simulink model "Engine_Propeller_Model_SAAM"  (R2018a)
settings: Solver=FixedStepAuto  StartTime=0.0  StopTime=10.0  FixedStep=dt  RelTol=1e-3
values from neighbouring files (symbols this model uses):
  dt = 0.05    [SmallAerobaticAirplaneModel.m]    (also in motorSpeedSS.m = 1; trim_airplane_min.m = 0.01)
  motorSpeed0 = 0    [SmallAerobaticAirplaneModel.m]    (also in create_engine_tables.m = fmincon(@(x)motorSpeedSS(x, Up, Vp, Wp, airDens, P_e_ic, vi0; trim_airplane_min.m = fmincon(@(x)motorSpeedSS(x, vcaso*cosd(aoadic), 0, -vcaso*si)
  vi0 = vcas(1)    [SmallAerobaticAirplaneModel.m]    (also in calculateThrustState.m = 0.001; create_engine_tables.m = fsolve(@(x)findVi2(x, vcaso*cosd(aoadic), 0, -vcaso*sind(aoa; findThrust.m = 0.01; trim_airplane_min.m = fsolve(@(x)findVi2(x, vcaso*cosd(aoadic), 0, -vcaso*sind(aoa)
settings Model: Creator=Kyle  LastModifiedBy=Kyle

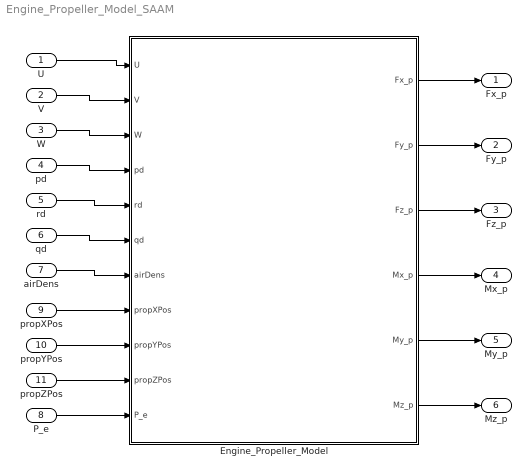
== system Engine_Propeller_Model_SAAM ==
  U : Inport
  V : Inport  Port=2
  W : Inport  Port=3
  pd : Inport  Port=4
  rd : Inport  Port=5
  qd : Inport  Port=6
  airDens : Inport  Port=7
  P_e : Inport  Port=8
  propXPos : Inport  Port=9
  propYPos : Inport  Port=10
  propZPos : Inport  Port=11
  Engine_Propeller_Model : Subsystem
  Fx_p : Outport
  Fy_p : Outport  Port=2
  Fz_p : Outport  Port=3
  Mx_p : Outport  Port=4
  My_p : Outport  Port=5
  Mz_p : Outport  Port=6
  wires:
  U/1 -> Engine_Propeller_Model/1(U)
  V/1 -> Engine_Propeller_Model/2(V)
  W/1 -> Engine_Propeller_Model/3(W)
  pd/1 -> Engine_Propeller_Model/4(pd)
  propXPos/1 -> Engine_Propeller_Model/8(propXPos)
  propYPos/1 -> Engine_Propeller_Model/9(propYPos)
  propZPos/1 -> Engine_Propeller_Model/10(propZPos)
  P_e/1 -> Engine_Propeller_Model/11(P_e)
  rd/1 -> Engine_Propeller_Model/5(rd)
  qd/1 -> Engine_Propeller_Model/6(qd)
  airDens/1 -> Engine_Propeller_Model/7(airDens)
  Engine_Propeller_Model/4(Mx_p) -> Mx_p/1
  Engine_Propeller_Model/6(Mz_p) -> Mz_p/1
  Engine_Propeller_Model/5(My_p) -> My_p/1
  Engine_Propeller_Model/2(Fy_p) -> Fy_p/1
  Engine_Propeller_Model/1(Fx_p) -> Fx_p/1
  Engine_Propeller_Model/3(Fz_p) -> Fz_p/1

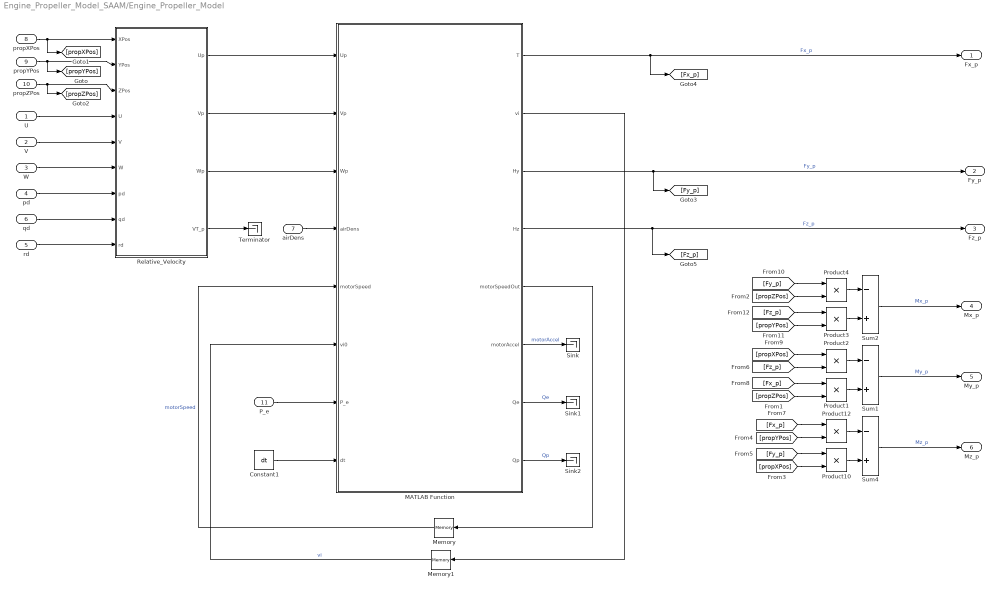
== system Engine_Propeller_Model_SAAM/Engine_Propeller_Model ==
  U : Inport
  V : Inport  Port=2
  W : Inport  Port=3
  pd : Inport  Port=4
  rd : Inport  Port=5
  qd : Inport  Port=6
  airDens : Inport  Port=7
  propXPos : Inport  Port=8
  propYPos : Inport  Port=9
  propZPos : Inport  Port=10
  P_e : Inport  Port=11
  Constant1 : Constant  Value=dt
  MATLAB Function : MATLAB Function  TreatAsAtomicUnit=on
  Memory : Memory  InitialCondition=motorSpeed0  LinearizeAsDelay=on
  Memory1 : Memory  InitialCondition=vi0  LinearizeAsDelay=on
  Product{1..4,10,12} (6 alike) : Product
  Relative_Velocity : Subsystem
  Sink : Terminator
  Sink1 : Terminator
  Sink2 : Terminator
  Sum1 : Sum  Inputs=-+
  Sum2 : Sum  Inputs=-+
  Sum4 : Sum  Inputs=-+
  Terminator : Terminator
  Fx_p : Outport
  Fy_p : Outport  Port=2
  Fz_p : Outport  Port=3
  Mx_p : Outport  Port=4
  My_p : Outport  Port=5
  Mz_p : Outport  Port=6
  wires:
  propYPos/1 -> [propYPos], Relative_Velocity/2(YPos)
  propZPos/1 -> [propZPos], Relative_Velocity/3(ZPos)
  U/1 -> Relative_Velocity/4(U)
  V/1 -> Relative_Velocity/5(V)
  W/1 -> Relative_Velocity/6(W)
  pd/1 -> Relative_Velocity/7(pd)
  rd/1 -> Relative_Velocity/9(rd)
  qd/1 -> Relative_Velocity/8(qd)
  propXPos/1 -> [propXPos], Relative_Velocity/1(XPos)
  [propZPos] -> Product1/2
  Product12/1 -> Sum4/1
  Sum4/1 -> Mz_p/1  "Mz_p"
  MATLAB Function/4(Hz) -> [Fz_p], Fz_p/1  "Fz_p"
  [propYPos] -> Product12/2
  Product10/1 -> Sum4/2
  [propXPos] -> Product10/2
  Relative_Velocity/4(VT_p) -> Terminator/1
  Relative_Velocity/1(Up) -> MATLAB Function/1(Up)
  Relative_Velocity/2(Vp) -> MATLAB Function/2(Vp)
  Relative_Velocity/3(Wp) -> MATLAB Function/3(Wp)
  airDens/1 -> MATLAB Function/4(airDens)
  MATLAB Function/5(motorSpeedOut) -> Memory/1
  Memory/1 -> MATLAB Function/5(motorSpeed)  "motorSpeed"
  MATLAB Function/2(vi) -> Memory1/1
  Memory1/1 -> MATLAB Function/6(vi0)  "vi"
  Constant1/1 -> MATLAB Function/8(dt)
  MATLAB Function/1(T) -> [Fx_p], Fx_p/1  "Fx_p"
  MATLAB Function/3(Hy) -> [Fy_p], Fy_p/1  "Fy_p"
  P_e/1 -> MATLAB Function/7(P_e)
  MATLAB Function/6(motorAccel) -> Sink/1  "motorAccel"
  MATLAB Function/7(Qe) -> Sink1/1  "Qe"
  MATLAB Function/8(Qp) -> Sink2/1  "Qp"
  [propZPos] -> Product4/2
  [Fy_p] -> Product10/1
  [Fx_p] -> Product12/1
  Product1/1 -> Sum1/2
  Product2/1 -> Sum1/1
  Sum1/1 -> My_p/1  "My_p"
  [Fx_p] -> Product1/1
  [Fz_p] -> Product2/2
  [propXPos] -> Product2/1
  Product4/1 -> Sum2/1
  Sum2/1 -> Mx_p/1  "Mx_p"
  Product3/1 -> Sum2/2
  [Fy_p] -> Product4/1
  [propYPos] -> Product3/2
  [Fz_p] -> Product3/1

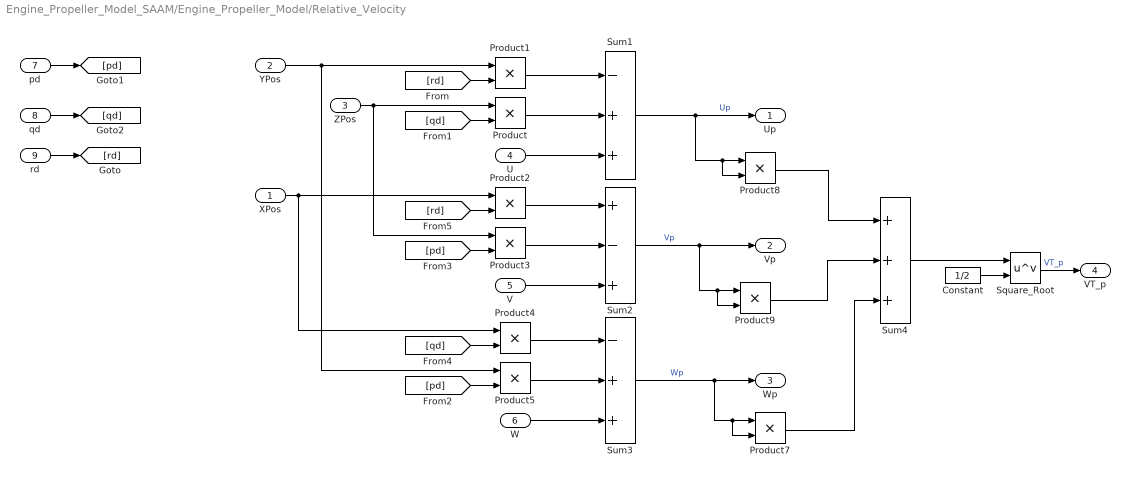
== system Engine_Propeller_Model_SAAM/Engine_Propeller_Model/Relative_Velocity ==
  XPos : Inport
  YPos : Inport  Port=2
  ZPos : Inport  Port=3
  U : Inport  Port=4
  V : Inport  Port=5
  W : Inport  Port=6
  pd : Inport  Port=7
  qd : Inport  Port=8
  rd : Inport  Port=9
  Constant : Constant  Value=1/2
  Product{,1..5,7..9} (9 alike) : Product
  Square_Root : Math  Operator=pow  SaturateOnIntegerOverflow=on
  Sum1 : Sum  Inputs=-++
  Sum2 : Sum  Inputs=+-+
  Sum3 : Sum  Inputs=-++
  Sum4 : Sum  Inputs=+++
  Up : Outport
  Vp : Outport  Port=2
  Wp : Outport  Port=3
  VT_p : Outport  Port=4
  wires:
  ZPos/1 -> Product3/1, Product/1
  Product/1 -> Sum1/2
  U/1 -> Sum1/3
  [rd] -> Product1/2
  Product1/1 -> Sum1/1
  rd/1 -> [rd]
  pd/1 -> [pd]
  qd/1 -> [qd]
  [qd] -> Product/2
  V/1 -> Sum2/3
  Sum3/1 -> Product7/2, Product7/1, Wp/1  "Wp"
  W/1 -> Sum3/3
  Product3/1 -> Sum2/2
  Product2/1 -> Sum2/1
  XPos/1 -> Product4/1, Product2/1
  YPos/1 -> Product5/1, Product1/1
  Product5/1 -> Sum3/2
  Product4/1 -> Sum3/1
  [pd] -> Product5/2
  [pd] -> Product3/2
  [rd] -> Product2/2
  [qd] -> Product4/2
  Sum1/1 -> Product8/2, Product8/1, Up/1  "Up"
  Sum2/1 -> Product9/1, Product9/2, Vp/1  "Vp"
  Square_Root/1 -> VT_p/1  "VT_p"
  Constant/1 -> Square_Root/2
  Sum4/1 -> Square_Root/1
  Product8/1 -> Sum4/1
  Product9/1 -> Sum4/2
  Product7/1 -> Sum4/3

== matlab function Engine_Propeller_Model_SAAM/Engine_Propeller_Model/MATLAB Function ==
  data: Up input double size=1; T output double size=1; Vp input double size=1; Wp input double size=1; airDens input double size=1; motorSpeed input double size=1; vi0 input double size=1; P_e input double size=1; vi output double size=1; Hy output double size=1; Hz output; motorSpeedOut output double size=1; dt input double size=1; motorAccel output; Qe output; Qp output
function [T, vi, Hy, Hz, motorSpeedOut, motorAccel, Qe, Qp] = calculateThrust(Up, Vp, Wp, airDens, motorSpeed, vi0, P_e, dt)
%UNTITLED Summary of this function goes here
%   Detailed explanation goes here

    coder.extrinsic('calculateThrustState')
    T = zeros(1,1);
    vi = zeros(1,1);
    Hy = zeros(1,1);
    Hz = zeros(1,1);
    motorSpeedOut = zeros(1,1);
    motorAccel = zeros(1,1);
    Qe = zeros(1,1);
    Qp = zeros(1,1);

    [T, vi, Hy, Hz, motorSpeedOut, motorAccel, Qe, Qp] = calculateThrustState(Up, Vp, Wp, airDens, motorSpeed, vi0, P_e, dt);

    
end
